simulink model "IndivdualProject4"  (R2021b)
settings: Solver=VariableStepAuto  StartTime=0.0  StopTime=inf  RelTol=1e-3
settings Model: Creator=davit  LastModifiedBy=minaebeid
settings SolverCC: AlgebraicLoopSolver=TrustRegion
settings DataIOCC: ReturnWorkspaceOutputs=off
settings DebuggingCC: SFMachineParentedDataDiag=warning  ArithmeticOperatorsInVariantConditions=warning
settings SFSimCC: SimUseLocalCustomCode=off  CustomCodeUndefinedFunction=UseInterfaceOnly
settings RTWCC: RTWUseLocalCustomCode=off

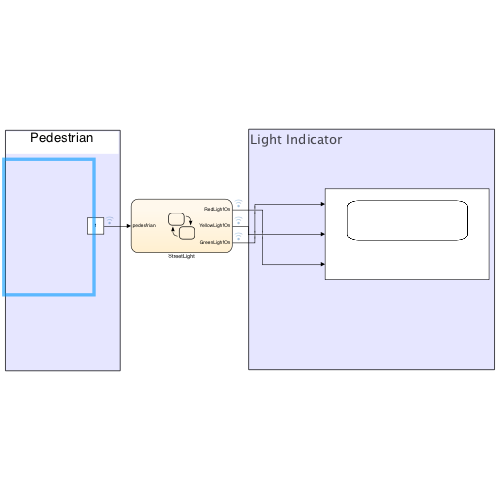
[thumbnail: Simulink's stored preview of the top-level diagram]
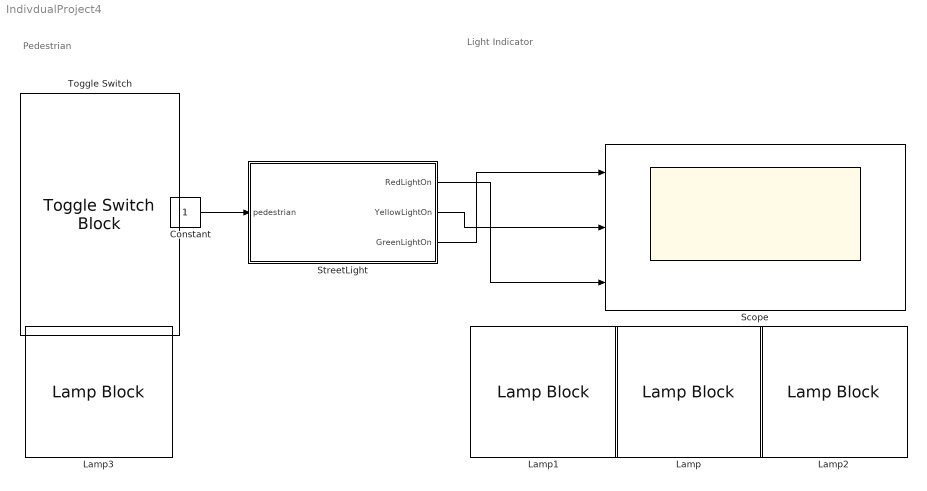
== system IndivdualProject4 ==
  note: Pedestrian
  note: Light Indicator
  Constant : Constant  OutDataTypeStr=boolean
  Lamp{,1..3} (4 alike) : LampBlock
  Scope : Scope  NumInputPorts=3
  StreetLight : Stateflow chart  TreatAsAtomicUnit=on
  Toggle Switch : ToggleSwitchBlock
      settings: Values={{'Off', 'On'}, [0 1]}
  wires:
  Constant/1 -> StreetLight/1(pedestrian)
  StreetLight/1(RedLightOn) -> Scope/3
  StreetLight/3(GreenLightOn) -> Scope/1
  StreetLight/2(YellowLightOn) -> Scope/2

== stateflow chart IndivdualProject4/StreetLight ==
  state Green
    GreenLightOn = 1;
    YellowLightOn = 0;
    RedLightOn = 0;
  state Red
    RedLightOn=1;
    YellowLightOn = 0;
    GreenLightOn = 0;
  state Pending
    GreenLightOn = 1;
    YellowLightOn = 0;
    RedLightOn = 0;
  state Yellow
    YellowLightOn=1;
    RedLightOn = 0;
    GreenLightOn = 0;
  Red -> Green : after(10, sec)
  Green -> Pending [order 2] : after(10, sec)[pedestrian == 1]
  Green -> Yellow [order 1] : after(10,sec)[pedestrian == 0]
  (default) -> Red
  Pending -> Yellow : after(10, sec)
  Yellow -> Red : after(3, sec)
  data: RedLightOn output; pedestrian input boolean =false; YellowLightOn output; GreenLightOn output
